simulink model "systolicArrayStreamOutput"  (R2021a)
settings: Solver=VariableStepAuto  StartTime=0.0  StopTime=13  RelTol=1e-3
libraries: hdlBasic x112, xbsIndex_r4 x1
settings Model: Creator=caval  LastModifiedBy=kv25

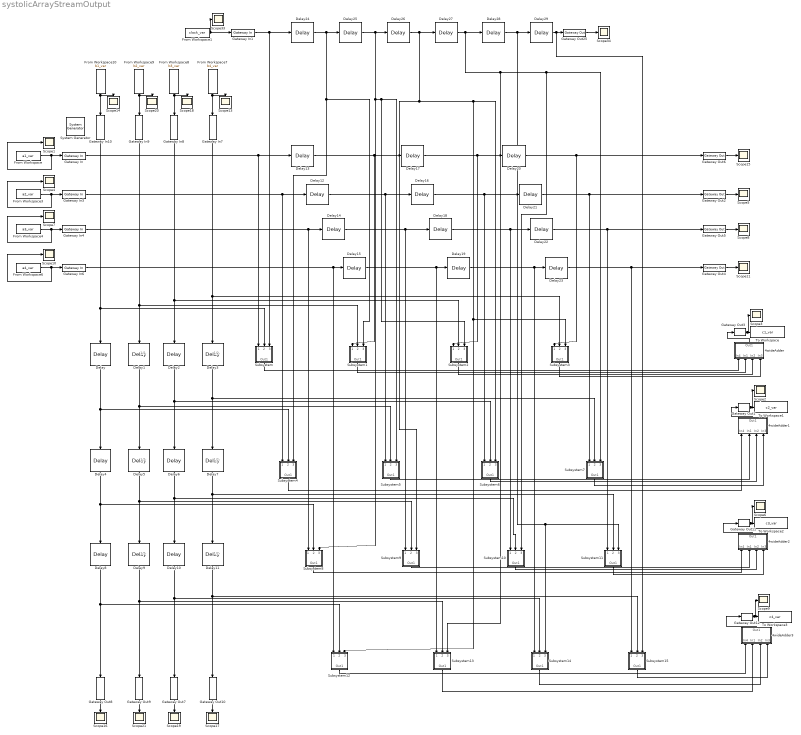
== system systolicArrayStreamOutput ==
  note: 1/2
  note: 1/2
  note: 1/2
  note: 1/2
  note: 1/2
  note: 1/2
  " System Generator" : xbsIndex_r4/ System Generator  Tag=genX  xilinxfamily=zynq  part=xc7z020  speed=-1  package=clg484  synthesis_tool=Vivado  clock_wrapper=Clock Enables  directory=./netlist2  proj_type=Vivado  Synth_file=Vivado Synthesis Defaults  Impl_file=Vivado Implementation Defaults  testbench=off  simulink_period=1  sysclk_period=10  dcm_input_clock_period=10  incr_netlist=off  trim_vbits=Everywhere in SubSystem  dbl_ovrd=According to Block Masks  core_generation=According to Block Masks  run_coregen=off  deprecated_control=off  eval_field=0  block_type=sysgen
  4wideAdder : Subsystem
  4wideAdder1 : Subsystem
  4wideAdder2 : Subsystem
  4wideAdder3 : Subsystem
  Delay{,1..29} (30 alike) : hdlBasic/Delay  rst=off  en=off  latency=1  reg_retiming=off  XmcBlockStatus=1  maskContainerNames=group1  block_type=delay  block_config=sysgen:Delay_config
  From Workspace : FromWorkspace  VariableName=a1_var
  From Workspace1 : FromWorkspace  VariableName=clock_var
  From Workspace10 : FromWorkspace  VariableName=b1_var
  From Workspace3 : FromWorkspace  VariableName=a2_var
  From Workspace4 : FromWorkspace  VariableName=a3_var
  From Workspace6 : FromWorkspace  VariableName=a4_var
  From Workspace7 : FromWorkspace  VariableName=b4_var
  From Workspace8 : FromWorkspace  VariableName=b3_var
  From Workspace9 : FromWorkspace  VariableName=b2_var
  Gateway In{,1,3..4,6..10} (9 alike) : hdlBasic/Gateway In  gui_display_data_type=Fixed-point  arith_type=Signed (2's comp)  n_bits=16  bin_pt=0  preci_type=Single  exp_width=8  frac_width=24  rows=1  columns=1  quantization="Round  (unbiased: +/- Inf)"  overflow=Saturate  period=1  UseAsADC=off  ADCChannel='1'  interface=None  automatic_assignment=on  address_offset=hex2dec('00')  intf_name=''  intf_description=''  default_value=0  timing_constraint=None  locs_specified=off  LOCs={}  io_standard={}  inherit_from_input=off  hdl_port=on  XmcBlockStatus=1  maskContainerNames=group4  block_type=gatewayin  block_config=sysgen:gateway_in_config  block_width_w=590  block_height_w=620  block_width=640  block_height=850
  Gateway Out{1..12,25} (13 alike) : hdlBasic/Gateway Out  inherit_from_input=off  hdl_port=on  rows=1  columns=1  UseAsDAC=off  DACChannel='1'  interface=None  automatic_assignment=on  address_offset=hex2dec('00')  intf_name=''  intf_description=''  timing_constraint=None  locs_specified=off  LOCs={}  io_standard={}  XmcBlockStatus=1  maskContainerNames=group4  block_type=gatewayout  block_config=sysgen:gateway_out_config  block_width_w=590  block_height_w=620  block_width=620  block_height=750
  Scope{1..11,13..21,33..34} (22 alike) : Scope
      Scope11 settings: Description=C14  AttributesFormatString=texttest
      Scope15 settings: Description=C14  AttributesFormatString=texttest
      Scope16 settings: Description=C14  AttributesFormatString=texttest
      Scope17 settings: Description=C14  AttributesFormatString=texttest
      Scope19 settings: Description=C14  AttributesFormatString=texttest
      Scope2 settings: Description=C14  AttributesFormatString=texttest
      Scope21 settings: Description=C14  AttributesFormatString=texttest
      Scope3 settings: Description=C14  AttributesFormatString=texttest
      Scope34 settings: Description=C14  AttributesFormatString=texttest
      Scope5 settings: Description=C14  AttributesFormatString=texttest
      Scope6 settings: Description=C14  AttributesFormatString=texttest
      Scope8 settings: Description=C14  AttributesFormatString=texttest
      Scope9 settings: Description=C14  AttributesFormatString=texttest
  Subsystem : Subsystem
  Subsystem1 : Subsystem
  Subsystem10 : Subsystem
  Subsystem11 : Subsystem
  Subsystem12 : Subsystem
  Subsystem13 : Subsystem
  Subsystem14 : Subsystem
  Subsystem15 : Subsystem
  Subsystem2 : Subsystem
  Subsystem3 : Subsystem
  Subsystem4 : Subsystem
  Subsystem5 : Subsystem
  Subsystem6 : Subsystem
  Subsystem7 : Subsystem
  Subsystem8 : Subsystem
  Subsystem9 : Subsystem
  To Workspace : ToWorkspace  VariableName=c1_var  SaveFormat=Timeseries  SampleTime=-1
  To Workspace1 : ToWorkspace  VariableName=c2_var  SaveFormat=Timeseries  SampleTime=-1
  To Workspace2 : ToWorkspace  VariableName=c3_var  SaveFormat=Timeseries  SampleTime=-1
  To Workspace3 : ToWorkspace  VariableName=c4_var  SaveFormat=Timeseries  SampleTime=-1
  wires:
  From Workspace/1 -> Scope1/1, Gateway In/1
  Gateway Out6/1 -> Scope15/1
  Gateway In/1 -> Delay13/1, Subsystem/1(In1)
  Gateway Out2/1 -> Scope5/1
  From Workspace3/1 -> Scope4/1, Gateway In3/1
  Gateway In3/1 -> Subsystem4/1(In1), Delay12/1
  From Workspace6/1 -> Scope10/1, Gateway In6/1
  Gateway Out5/1 -> Scope8/1
  Gateway Out4/1 -> Scope11/1
  From Workspace4/1 -> Scope7/1, Gateway In4/1
  Gateway In6/1 -> Subsystem12/1(In1), Delay15/1
  Gateway In4/1 -> Subsystem8/1(In1), Delay14/1
  From Workspace8/1 -> Scope18/1, Gateway In8/1
  Gateway Out7/1 -> Scope19/1
  Gateway In9/1 -> Subsystem1/2(In2), Delay1/1
  Gateway In10/1 -> Subsystem/2(In2), Delay/1
  Gateway Out8/1 -> Scope16/1
  From Workspace10/1 -> Scope14/1, Gateway In10/1
  Gateway Out10/1 -> Scope17/1
  From Workspace9/1 -> Scope20/1, Gateway In9/1
  Gateway Out9/1 -> Scope21/1
  From Workspace7/1 -> Scope13/1, Gateway In7/1
  Gateway In8/1 -> Subsystem2/2(In2), Delay2/1
  Gateway In7/1 -> Subsystem3/2(In2), Delay3/1
  Delay/1 -> Subsystem4/2(In2), Delay4/1
  Delay4/1 -> Subsystem8/2(In2), Delay8/1
  Delay13/1 -> Subsystem1/1(In1), Delay17/1
  Delay12/1 -> Delay16/1, Subsystem5/1(In1)
  Delay1/1 -> Subsystem5/2(In2), Delay5/1
  Delay2/1 -> Subsystem6/2(In2), Delay6/1
  Delay3/1 -> Subsystem7/2(In2), Delay7/1
  Delay5/1 -> Subsystem9/2(In2), Delay9/1
  Delay6/1 -> Subsystem10/2(In2), Delay10/1
  Delay7/1 -> Subsystem11/2(In2), Delay11/1
  Delay20/1 -> Subsystem3/1(In1), Gateway Out6/1
  Delay16/1 -> Subsystem6/1(In1), Delay21/1
  Delay21/1 -> Subsystem7/1(In1), Gateway Out2/1
  Delay8/1 -> Subsystem12/2(In2), Gateway Out8/1
  Delay11/1 -> Subsystem15/2(In2), Gateway Out10/1
  Delay9/1 -> Subsystem13/2(In2), Gateway Out9/1
  Delay10/1 -> Subsystem14/2(In2), Gateway Out7/1
  Delay18/1 -> Subsystem10/1(In1), Delay22/1
  Delay22/1 -> Subsystem11/1(In1), Gateway Out5/1
  Delay19/1 -> Subsystem14/1(In1), Delay23/1
  Delay23/1 -> Subsystem15/1(In1), Gateway Out4/1
  Delay14/1 -> Subsystem9/1(In1), Delay18/1
  Delay15/1 -> Subsystem13/1(In1), Delay19/1
  Delay17/1 -> Subsystem2/1(In1), Delay20/1
  From Workspace1/1 -> Scope33/1, Gateway In1/1
  Gateway In1/1 -> Subsystem/3(In3), Delay24/1
  Delay24/1 -> Subsystem4/3(In3), Subsystem1/3(In3), Delay25/1
  Delay25/1 -> Subsystem8/3(In3), Subsystem5/3(In3), Subsystem2/3(In3), Delay26/1
  Delay28/1 -> Delay29/1, Subsystem14/3(In3), Subsystem11/3(In3)
  Delay27/1 -> Subsystem13/3(In3), Subsystem10/3(In3), Subsystem7/3(In3), Delay28/1
  Gateway Out25/1 -> Scope34/1
  Delay29/1 -> Subsystem15/3(In3), Gateway Out25/1
  Delay26/1 -> Subsystem9/3(In3), Subsystem6/3(In3), Subsystem12/3(In3), Subsystem3/3(In3), Delay27/1
  4wideAdder/1(Out1) -> Gateway Out3/1
  Gateway Out3/1 -> Scope3/1, To Workspace/1
  Subsystem1/1(Out1) -> 4wideAdder/2(In1)
  Subsystem2/1(Out1) -> 4wideAdder/3(In2)
  Subsystem3/1(Out1) -> 4wideAdder/4(In3)
  Subsystem4/1(Out1) -> 4wideAdder1/1(In4)
  Subsystem5/1(Out1) -> 4wideAdder1/2(In1)
  Subsystem6/1(Out1) -> 4wideAdder1/3(In2)
  Subsystem7/1(Out1) -> 4wideAdder1/4(In3)
  Subsystem8/1(Out1) -> 4wideAdder2/1(In4)
  Subsystem9/1(Out1) -> 4wideAdder2/2(In1)
  Subsystem10/1(Out1) -> 4wideAdder2/3(In2)
  Subsystem11/1(Out1) -> 4wideAdder2/4(In3)
  Subsystem12/1(Out1) -> 4wideAdder3/1(In4)
  Subsystem13/1(Out1) -> 4wideAdder3/2(In1)
  Subsystem14/1(Out1) -> 4wideAdder3/3(In2)
  Subsystem15/1(Out1) -> 4wideAdder3/4(In3)
  Subsystem/1(Out1) -> 4wideAdder/1(In4)
  4wideAdder1/1(Out1) -> Gateway Out1/1
  Gateway Out1/1 -> Scope2/1, To Workspace1/1
  4wideAdder2/1(Out1) -> Gateway Out11/1
  Gateway Out11/1 -> Scope6/1, To Workspace2/1
  4wideAdder3/1(Out1) -> Gateway Out12/1
  Gateway Out12/1 -> Scope9/1, To Workspace3/1

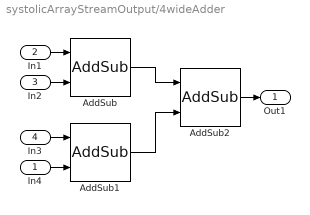
== system systolicArrayStreamOutput/4wideAdder ==
  In4 : Inport
  In1 : Inport  Port=2
  In2 : Inport  Port=3
  In3 : Inport  Port=4
  AddSub : hdlBasic/AddSub  mode=Addition  use_carryin=off  use_carryout=off  en=off  latency=0  precision=Full  arith_type=Unsigned  n_bits=16  bin_pt=14  quantization=Truncate  overflow=Wrap  use_behavioral_HDL=off  hw_selection=Fabric  pipelined=off  XmcBlockStatus=1  maskContainerNames=tabcontainer1  block_type=addsub  block_config=sysgen:Addsub_config
  AddSub1 : hdlBasic/AddSub  mode=Addition  use_carryin=off  use_carryout=off  en=off  latency=0  precision=Full  arith_type=Unsigned  n_bits=16  bin_pt=14  quantization=Truncate  overflow=Wrap  use_behavioral_HDL=off  hw_selection=Fabric  pipelined=off  XmcBlockStatus=1  maskContainerNames=tabcontainer1  block_type=addsub  block_config=sysgen:Addsub_config
  AddSub2 : hdlBasic/AddSub  mode=Addition  use_carryin=off  use_carryout=off  en=off  latency=0  precision=Full  arith_type=Unsigned  n_bits=16  bin_pt=14  quantization=Truncate  overflow=Wrap  use_behavioral_HDL=off  hw_selection=Fabric  pipelined=off  XmcBlockStatus=1  maskContainerNames=tabcontainer1  block_type=addsub  block_config=sysgen:Addsub_config
  Out1 : Outport
  wires:
  In1/1 -> AddSub/1
  AddSub1/1 -> AddSub2/2
  AddSub/1 -> AddSub2/1
  In4/1 -> AddSub1/2
  In3/1 -> AddSub1/1
  AddSub2/1 -> Out1/1
  In2/1 -> AddSub/2

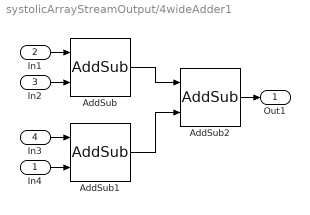
== system systolicArrayStreamOutput/4wideAdder1 ==
  In4 : Inport
  In1 : Inport  Port=2
  In2 : Inport  Port=3
  In3 : Inport  Port=4
  AddSub : hdlBasic/AddSub  mode=Addition  use_carryin=off  use_carryout=off  en=off  latency=0  precision=Full  arith_type=Unsigned  n_bits=16  bin_pt=14  quantization=Truncate  overflow=Wrap  use_behavioral_HDL=off  hw_selection=Fabric  pipelined=off  XmcBlockStatus=1  maskContainerNames=tabcontainer1  block_type=addsub  block_config=sysgen:Addsub_config
  AddSub1 : hdlBasic/AddSub  mode=Addition  use_carryin=off  use_carryout=off  en=off  latency=0  precision=Full  arith_type=Unsigned  n_bits=16  bin_pt=14  quantization=Truncate  overflow=Wrap  use_behavioral_HDL=off  hw_selection=Fabric  pipelined=off  XmcBlockStatus=1  maskContainerNames=tabcontainer1  block_type=addsub  block_config=sysgen:Addsub_config
  AddSub2 : hdlBasic/AddSub  mode=Addition  use_carryin=off  use_carryout=off  en=off  latency=0  precision=Full  arith_type=Unsigned  n_bits=16  bin_pt=14  quantization=Truncate  overflow=Wrap  use_behavioral_HDL=off  hw_selection=Fabric  pipelined=off  XmcBlockStatus=1  maskContainerNames=tabcontainer1  block_type=addsub  block_config=sysgen:Addsub_config
  Out1 : Outport
  wires:
  In1/1 -> AddSub/1
  AddSub1/1 -> AddSub2/2
  AddSub/1 -> AddSub2/1
  In4/1 -> AddSub1/2
  In3/1 -> AddSub1/1
  AddSub2/1 -> Out1/1
  In2/1 -> AddSub/2

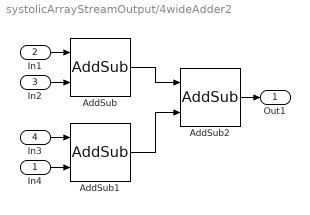
== system systolicArrayStreamOutput/4wideAdder2 ==
  In4 : Inport
  In1 : Inport  Port=2
  In2 : Inport  Port=3
  In3 : Inport  Port=4
  AddSub : hdlBasic/AddSub  mode=Addition  use_carryin=off  use_carryout=off  en=off  latency=0  precision=Full  arith_type=Unsigned  n_bits=16  bin_pt=14  quantization=Truncate  overflow=Wrap  use_behavioral_HDL=off  hw_selection=Fabric  pipelined=off  XmcBlockStatus=1  maskContainerNames=tabcontainer1  block_type=addsub  block_config=sysgen:Addsub_config
  AddSub1 : hdlBasic/AddSub  mode=Addition  use_carryin=off  use_carryout=off  en=off  latency=0  precision=Full  arith_type=Unsigned  n_bits=16  bin_pt=14  quantization=Truncate  overflow=Wrap  use_behavioral_HDL=off  hw_selection=Fabric  pipelined=off  XmcBlockStatus=1  maskContainerNames=tabcontainer1  block_type=addsub  block_config=sysgen:Addsub_config
  AddSub2 : hdlBasic/AddSub  mode=Addition  use_carryin=off  use_carryout=off  en=off  latency=0  precision=Full  arith_type=Unsigned  n_bits=16  bin_pt=14  quantization=Truncate  overflow=Wrap  use_behavioral_HDL=off  hw_selection=Fabric  pipelined=off  XmcBlockStatus=1  maskContainerNames=tabcontainer1  block_type=addsub  block_config=sysgen:Addsub_config
  Out1 : Outport
  wires:
  In1/1 -> AddSub/1
  AddSub1/1 -> AddSub2/2
  AddSub/1 -> AddSub2/1
  In4/1 -> AddSub1/2
  In3/1 -> AddSub1/1
  AddSub2/1 -> Out1/1
  In2/1 -> AddSub/2

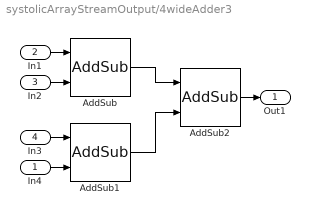
== system systolicArrayStreamOutput/4wideAdder3 ==
  In4 : Inport
  In1 : Inport  Port=2
  In2 : Inport  Port=3
  In3 : Inport  Port=4
  AddSub : hdlBasic/AddSub  mode=Addition  use_carryin=off  use_carryout=off  en=off  latency=0  precision=Full  arith_type=Unsigned  n_bits=16  bin_pt=14  quantization=Truncate  overflow=Wrap  use_behavioral_HDL=off  hw_selection=Fabric  pipelined=off  XmcBlockStatus=1  maskContainerNames=tabcontainer1  block_type=addsub  block_config=sysgen:Addsub_config
  AddSub1 : hdlBasic/AddSub  mode=Addition  use_carryin=off  use_carryout=off  en=off  latency=0  precision=Full  arith_type=Unsigned  n_bits=16  bin_pt=14  quantization=Truncate  overflow=Wrap  use_behavioral_HDL=off  hw_selection=Fabric  pipelined=off  XmcBlockStatus=1  maskContainerNames=tabcontainer1  block_type=addsub  block_config=sysgen:Addsub_config
  AddSub2 : hdlBasic/AddSub  mode=Addition  use_carryin=off  use_carryout=off  en=off  latency=0  precision=Full  arith_type=Unsigned  n_bits=16  bin_pt=14  quantization=Truncate  overflow=Wrap  use_behavioral_HDL=off  hw_selection=Fabric  pipelined=off  XmcBlockStatus=1  maskContainerNames=tabcontainer1  block_type=addsub  block_config=sysgen:Addsub_config
  Out1 : Outport
  wires:
  In1/1 -> AddSub/1
  AddSub1/1 -> AddSub2/2
  AddSub/1 -> AddSub2/1
  In4/1 -> AddSub1/2
  In3/1 -> AddSub1/1
  AddSub2/1 -> Out1/1
  In2/1 -> AddSub/2

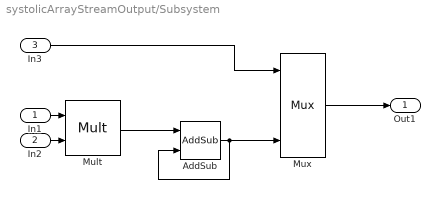
== system systolicArrayStreamOutput/Subsystem ==
  In1 : Inport
  In2 : Inport  Port=2
  In3 : Inport  Port=3
  AddSub : hdlBasic/AddSub  mode=Addition  use_carryin=off  use_carryout=off  en=off  latency=1  precision=User Defined  arith_type=Unsigned  n_bits=16  bin_pt=0  quantization=Truncate  overflow=Wrap  use_behavioral_HDL=off  hw_selection=Fabric  pipelined=off  XmcBlockStatus=1  maskContainerNames=tabcontainer1  block_type=addsub  block_config=sysgen:Addsub_config
  Mult : hdlBasic/Mult  precision=Full  arith_type="Signed  (2's comp)"  n_bits=16  bin_pt=14  quantization=Truncate  overflow=Wrap  en=off  latency=0  use_behavioral_HDL=off  opt=Speed  use_embedded=on  optimum_pipeline=off  pipeline=on  use_rpm=on  placement_style=Triangular  XmcBlockStatus=1  maskContainerNames=group1  block_type=mult  block_config=sysgen:Mult_config
  Mux : hdlBasic/Mux  inputs=2  en=off  latency=1  precision=Full  arith_type=Unsigned  n_bits=16  bin_pt=14  quantization=Truncate  overflow=Wrap  XmcBlockStatus=1  maskContainerNames=tabcontainer1  block_type=mux  block_config=sysgen:Mux_config
  Out1 : Outport
  wires:
  In1/1 -> Mult/1
  AddSub/1 -> Mux/3, AddSub/2
  In2/1 -> Mult/2
  Mult/1 -> AddSub/1
  In3/1 -> Mux/1
  Mux/1 -> Out1/1

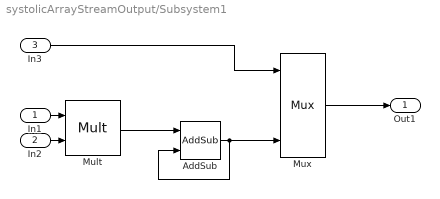
== system systolicArrayStreamOutput/Subsystem1 ==
  In1 : Inport
  In2 : Inport  Port=2
  In3 : Inport  Port=3
  AddSub : hdlBasic/AddSub  mode=Addition  use_carryin=off  use_carryout=off  en=off  latency=1  precision=User Defined  arith_type=Unsigned  n_bits=16  bin_pt=0  quantization=Truncate  overflow=Wrap  use_behavioral_HDL=off  hw_selection=Fabric  pipelined=off  XmcBlockStatus=1  maskContainerNames=tabcontainer1  block_type=addsub  block_config=sysgen:Addsub_config
  Mult : hdlBasic/Mult  precision=Full  arith_type="Signed  (2's comp)"  n_bits=16  bin_pt=14  quantization=Truncate  overflow=Wrap  en=off  latency=0  use_behavioral_HDL=off  opt=Speed  use_embedded=on  optimum_pipeline=off  pipeline=on  use_rpm=on  placement_style=Triangular  XmcBlockStatus=1  maskContainerNames=group1  block_type=mult  block_config=sysgen:Mult_config
  Mux : hdlBasic/Mux  inputs=2  en=off  latency=1  precision=Full  arith_type=Unsigned  n_bits=16  bin_pt=14  quantization=Truncate  overflow=Wrap  XmcBlockStatus=1  maskContainerNames=tabcontainer1  block_type=mux  block_config=sysgen:Mux_config
  Out1 : Outport
  wires:
  In1/1 -> Mult/1
  AddSub/1 -> Mux/3, AddSub/2
  In2/1 -> Mult/2
  Mult/1 -> AddSub/1
  In3/1 -> Mux/1
  Mux/1 -> Out1/1

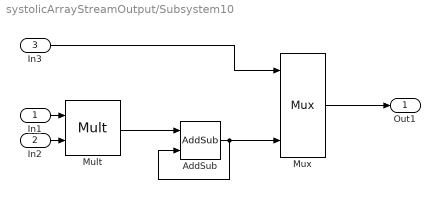
== system systolicArrayStreamOutput/Subsystem10 ==
  In1 : Inport
  In2 : Inport  Port=2
  In3 : Inport  Port=3
  AddSub : hdlBasic/AddSub  mode=Addition  use_carryin=off  use_carryout=off  en=off  latency=1  precision=User Defined  arith_type=Unsigned  n_bits=16  bin_pt=0  quantization=Truncate  overflow=Wrap  use_behavioral_HDL=off  hw_selection=Fabric  pipelined=off  XmcBlockStatus=1  maskContainerNames=tabcontainer1  block_type=addsub  block_config=sysgen:Addsub_config
  Mult : hdlBasic/Mult  precision=Full  arith_type="Signed  (2's comp)"  n_bits=16  bin_pt=14  quantization=Truncate  overflow=Wrap  en=off  latency=0  use_behavioral_HDL=off  opt=Speed  use_embedded=on  optimum_pipeline=off  pipeline=on  use_rpm=on  placement_style=Triangular  XmcBlockStatus=1  maskContainerNames=group1  block_type=mult  block_config=sysgen:Mult_config
  Mux : hdlBasic/Mux  inputs=2  en=off  latency=1  precision=Full  arith_type=Unsigned  n_bits=16  bin_pt=14  quantization=Truncate  overflow=Wrap  XmcBlockStatus=1  maskContainerNames=tabcontainer1  block_type=mux  block_config=sysgen:Mux_config
  Out1 : Outport
  wires:
  In1/1 -> Mult/1
  AddSub/1 -> Mux/3, AddSub/2
  In2/1 -> Mult/2
  Mult/1 -> AddSub/1
  In3/1 -> Mux/1
  Mux/1 -> Out1/1

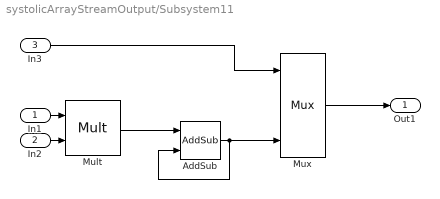
== system systolicArrayStreamOutput/Subsystem11 ==
  In1 : Inport
  In2 : Inport  Port=2
  In3 : Inport  Port=3
  AddSub : hdlBasic/AddSub  mode=Addition  use_carryin=off  use_carryout=off  en=off  latency=1  precision=User Defined  arith_type=Unsigned  n_bits=16  bin_pt=0  quantization=Truncate  overflow=Wrap  use_behavioral_HDL=off  hw_selection=Fabric  pipelined=off  XmcBlockStatus=1  maskContainerNames=tabcontainer1  block_type=addsub  block_config=sysgen:Addsub_config
  Mult : hdlBasic/Mult  precision=Full  arith_type="Signed  (2's comp)"  n_bits=16  bin_pt=14  quantization=Truncate  overflow=Wrap  en=off  latency=0  use_behavioral_HDL=off  opt=Speed  use_embedded=on  optimum_pipeline=off  pipeline=on  use_rpm=on  placement_style=Triangular  XmcBlockStatus=1  maskContainerNames=group1  block_type=mult  block_config=sysgen:Mult_config
  Mux : hdlBasic/Mux  inputs=2  en=off  latency=1  precision=Full  arith_type=Unsigned  n_bits=16  bin_pt=14  quantization=Truncate  overflow=Wrap  XmcBlockStatus=1  maskContainerNames=tabcontainer1  block_type=mux  block_config=sysgen:Mux_config
  Out1 : Outport
  wires:
  In1/1 -> Mult/1
  AddSub/1 -> Mux/3, AddSub/2
  In2/1 -> Mult/2
  Mult/1 -> AddSub/1
  In3/1 -> Mux/1
  Mux/1 -> Out1/1

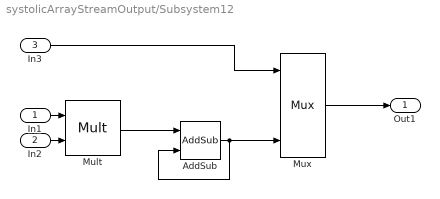
== system systolicArrayStreamOutput/Subsystem12 ==
  In1 : Inport
  In2 : Inport  Port=2
  In3 : Inport  Port=3
  AddSub : hdlBasic/AddSub  mode=Addition  use_carryin=off  use_carryout=off  en=off  latency=1  precision=User Defined  arith_type=Unsigned  n_bits=16  bin_pt=0  quantization=Truncate  overflow=Wrap  use_behavioral_HDL=off  hw_selection=Fabric  pipelined=off  XmcBlockStatus=1  maskContainerNames=tabcontainer1  block_type=addsub  block_config=sysgen:Addsub_config
  Mult : hdlBasic/Mult  precision=Full  arith_type="Signed  (2's comp)"  n_bits=16  bin_pt=14  quantization=Truncate  overflow=Wrap  en=off  latency=0  use_behavioral_HDL=off  opt=Speed  use_embedded=on  optimum_pipeline=off  pipeline=on  use_rpm=on  placement_style=Triangular  XmcBlockStatus=1  maskContainerNames=group1  block_type=mult  block_config=sysgen:Mult_config
  Mux : hdlBasic/Mux  inputs=2  en=off  latency=1  precision=Full  arith_type=Unsigned  n_bits=16  bin_pt=14  quantization=Truncate  overflow=Wrap  XmcBlockStatus=1  maskContainerNames=tabcontainer1  block_type=mux  block_config=sysgen:Mux_config
  Out1 : Outport
  wires:
  In1/1 -> Mult/1
  AddSub/1 -> Mux/3, AddSub/2
  In2/1 -> Mult/2
  Mult/1 -> AddSub/1
  In3/1 -> Mux/1
  Mux/1 -> Out1/1

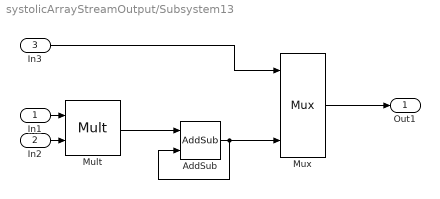
== system systolicArrayStreamOutput/Subsystem13 ==
  In1 : Inport
  In2 : Inport  Port=2
  In3 : Inport  Port=3
  AddSub : hdlBasic/AddSub  mode=Addition  use_carryin=off  use_carryout=off  en=off  latency=1  precision=User Defined  arith_type=Unsigned  n_bits=16  bin_pt=0  quantization=Truncate  overflow=Wrap  use_behavioral_HDL=off  hw_selection=Fabric  pipelined=off  XmcBlockStatus=1  maskContainerNames=tabcontainer1  block_type=addsub  block_config=sysgen:Addsub_config
  Mult : hdlBasic/Mult  precision=Full  arith_type="Signed  (2's comp)"  n_bits=16  bin_pt=14  quantization=Truncate  overflow=Wrap  en=off  latency=0  use_behavioral_HDL=off  opt=Speed  use_embedded=on  optimum_pipeline=off  pipeline=on  use_rpm=on  placement_style=Triangular  XmcBlockStatus=1  maskContainerNames=group1  block_type=mult  block_config=sysgen:Mult_config
  Mux : hdlBasic/Mux  inputs=2  en=off  latency=1  precision=Full  arith_type=Unsigned  n_bits=16  bin_pt=14  quantization=Truncate  overflow=Wrap  XmcBlockStatus=1  maskContainerNames=tabcontainer1  block_type=mux  block_config=sysgen:Mux_config
  Out1 : Outport
  wires:
  In1/1 -> Mult/1
  AddSub/1 -> Mux/3, AddSub/2
  In2/1 -> Mult/2
  Mult/1 -> AddSub/1
  In3/1 -> Mux/1
  Mux/1 -> Out1/1

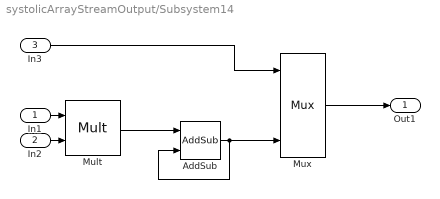
== system systolicArrayStreamOutput/Subsystem14 ==
  In1 : Inport
  In2 : Inport  Port=2
  In3 : Inport  Port=3
  AddSub : hdlBasic/AddSub  mode=Addition  use_carryin=off  use_carryout=off  en=off  latency=1  precision=User Defined  arith_type=Unsigned  n_bits=16  bin_pt=0  quantization=Truncate  overflow=Wrap  use_behavioral_HDL=off  hw_selection=Fabric  pipelined=off  XmcBlockStatus=1  maskContainerNames=tabcontainer1  block_type=addsub  block_config=sysgen:Addsub_config
  Mult : hdlBasic/Mult  precision=Full  arith_type="Signed  (2's comp)"  n_bits=16  bin_pt=14  quantization=Truncate  overflow=Wrap  en=off  latency=0  use_behavioral_HDL=off  opt=Speed  use_embedded=on  optimum_pipeline=off  pipeline=on  use_rpm=on  placement_style=Triangular  XmcBlockStatus=1  maskContainerNames=group1  block_type=mult  block_config=sysgen:Mult_config
  Mux : hdlBasic/Mux  inputs=2  en=off  latency=1  precision=Full  arith_type=Unsigned  n_bits=16  bin_pt=14  quantization=Truncate  overflow=Wrap  XmcBlockStatus=1  maskContainerNames=tabcontainer1  block_type=mux  block_config=sysgen:Mux_config
  Out1 : Outport
  wires:
  In1/1 -> Mult/1
  AddSub/1 -> Mux/3, AddSub/2
  In2/1 -> Mult/2
  Mult/1 -> AddSub/1
  In3/1 -> Mux/1
  Mux/1 -> Out1/1

== system systolicArrayStreamOutput/Subsystem15 ==
  In1 : Inport
  In2 : Inport  Port=2
  In3 : Inport  Port=3
  AddSub : hdlBasic/AddSub  mode=Addition  use_carryin=off  use_carryout=off  en=off  latency=1  precision=User Defined  arith_type=Unsigned  n_bits=16  bin_pt=0  quantization=Truncate  overflow=Wrap  use_behavioral_HDL=off  hw_selection=Fabric  pipelined=off  XmcBlockStatus=1  maskContainerNames=tabcontainer1  block_type=addsub  block_config=sysgen:Addsub_config
  Mult : hdlBasic/Mult  precision=Full  arith_type="Signed  (2's comp)"  n_bits=16  bin_pt=14  quantization=Truncate  overflow=Wrap  en=off  latency=0  use_behavioral_HDL=off  opt=Speed  use_embedded=on  optimum_pipeline=off  pipeline=on  use_rpm=on  placement_style=Triangular  XmcBlockStatus=1  maskContainerNames=group1  block_type=mult  block_config=sysgen:Mult_config
  Mux : hdlBasic/Mux  inputs=2  en=off  latency=1  precision=Full  arith_type=Unsigned  n_bits=16  bin_pt=14  quantization=Truncate  overflow=Wrap  XmcBlockStatus=1  maskContainerNames=tabcontainer1  block_type=mux  block_config=sysgen:Mux_config
  Out1 : Outport
  wires:
  In1/1 -> Mult/1
  AddSub/1 -> Mux/3, AddSub/2
  In2/1 -> Mult/2
  Mult/1 -> AddSub/1
  In3/1 -> Mux/1
  Mux/1 -> Out1/1

== system systolicArrayStreamOutput/Subsystem2 ==
  In1 : Inport
  In2 : Inport  Port=2
  In3 : Inport  Port=3
  AddSub : hdlBasic/AddSub  mode=Addition  use_carryin=off  use_carryout=off  en=off  latency=1  precision=User Defined  arith_type=Unsigned  n_bits=16  bin_pt=0  quantization=Truncate  overflow=Wrap  use_behavioral_HDL=off  hw_selection=Fabric  pipelined=off  XmcBlockStatus=1  maskContainerNames=tabcontainer1  block_type=addsub  block_config=sysgen:Addsub_config
  Mult : hdlBasic/Mult  precision=Full  arith_type="Signed  (2's comp)"  n_bits=16  bin_pt=14  quantization=Truncate  overflow=Wrap  en=off  latency=0  use_behavioral_HDL=off  opt=Speed  use_embedded=on  optimum_pipeline=off  pipeline=on  use_rpm=on  placement_style=Triangular  XmcBlockStatus=1  maskContainerNames=group1  block_type=mult  block_config=sysgen:Mult_config
  Mux : hdlBasic/Mux  inputs=2  en=off  latency=1  precision=Full  arith_type=Unsigned  n_bits=16  bin_pt=14  quantization=Truncate  overflow=Wrap  XmcBlockStatus=1  maskContainerNames=tabcontainer1  block_type=mux  block_config=sysgen:Mux_config
  Out1 : Outport
  wires:
  In1/1 -> Mult/1
  AddSub/1 -> Mux/3, AddSub/2
  In2/1 -> Mult/2
  Mult/1 -> AddSub/1
  In3/1 -> Mux/1
  Mux/1 -> Out1/1

== system systolicArrayStreamOutput/Subsystem3 ==
  In1 : Inport
  In2 : Inport  Port=2
  In3 : Inport  Port=3
  AddSub : hdlBasic/AddSub  mode=Addition  use_carryin=off  use_carryout=off  en=off  latency=1  precision=User Defined  arith_type=Unsigned  n_bits=16  bin_pt=0  quantization=Truncate  overflow=Wrap  use_behavioral_HDL=off  hw_selection=Fabric  pipelined=off  XmcBlockStatus=1  maskContainerNames=tabcontainer1  block_type=addsub  block_config=sysgen:Addsub_config
  Mult : hdlBasic/Mult  precision=Full  arith_type="Signed  (2's comp)"  n_bits=16  bin_pt=14  quantization=Truncate  overflow=Wrap  en=off  latency=0  use_behavioral_HDL=off  opt=Speed  use_embedded=on  optimum_pipeline=off  pipeline=on  use_rpm=on  placement_style=Triangular  XmcBlockStatus=1  maskContainerNames=group1  block_type=mult  block_config=sysgen:Mult_config
  Mux : hdlBasic/Mux  inputs=2  en=off  latency=1  precision=Full  arith_type=Unsigned  n_bits=16  bin_pt=14  quantization=Truncate  overflow=Wrap  XmcBlockStatus=1  maskContainerNames=tabcontainer1  block_type=mux  block_config=sysgen:Mux_config
  Out1 : Outport
  wires:
  In1/1 -> Mult/1
  AddSub/1 -> Mux/3, AddSub/2
  In2/1 -> Mult/2
  Mult/1 -> AddSub/1
  In3/1 -> Mux/1
  Mux/1 -> Out1/1

== system systolicArrayStreamOutput/Subsystem4 ==
  In1 : Inport
  In2 : Inport  Port=2
  In3 : Inport  Port=3
  AddSub : hdlBasic/AddSub  mode=Addition  use_carryin=off  use_carryout=off  en=off  latency=1  precision=User Defined  arith_type=Unsigned  n_bits=16  bin_pt=0  quantization=Truncate  overflow=Wrap  use_behavioral_HDL=off  hw_selection=Fabric  pipelined=off  XmcBlockStatus=1  maskContainerNames=tabcontainer1  block_type=addsub  block_config=sysgen:Addsub_config
  Mult : hdlBasic/Mult  precision=Full  arith_type="Signed  (2's comp)"  n_bits=16  bin_pt=14  quantization=Truncate  overflow=Wrap  en=off  latency=0  use_behavioral_HDL=off  opt=Speed  use_embedded=on  optimum_pipeline=off  pipeline=on  use_rpm=on  placement_style=Triangular  XmcBlockStatus=1  maskContainerNames=group1  block_type=mult  block_config=sysgen:Mult_config
  Mux : hdlBasic/Mux  inputs=2  en=off  latency=1  precision=Full  arith_type=Unsigned  n_bits=16  bin_pt=14  quantization=Truncate  overflow=Wrap  XmcBlockStatus=1  maskContainerNames=tabcontainer1  block_type=mux  block_config=sysgen:Mux_config
  Out1 : Outport
  wires:
  In1/1 -> Mult/1
  AddSub/1 -> Mux/3, AddSub/2
  In2/1 -> Mult/2
  Mult/1 -> AddSub/1
  In3/1 -> Mux/1
  Mux/1 -> Out1/1

== system systolicArrayStreamOutput/Subsystem5 ==
  In1 : Inport
  In2 : Inport  Port=2
  In3 : Inport  Port=3
  AddSub : hdlBasic/AddSub  mode=Addition  use_carryin=off  use_carryout=off  en=off  latency=1  precision=User Defined  arith_type=Unsigned  n_bits=16  bin_pt=0  quantization=Truncate  overflow=Wrap  use_behavioral_HDL=off  hw_selection=Fabric  pipelined=off  XmcBlockStatus=1  maskContainerNames=tabcontainer1  block_type=addsub  block_config=sysgen:Addsub_config
  Mult : hdlBasic/Mult  precision=Full  arith_type="Signed  (2's comp)"  n_bits=16  bin_pt=14  quantization=Truncate  overflow=Wrap  en=off  latency=0  use_behavioral_HDL=off  opt=Speed  use_embedded=on  optimum_pipeline=off  pipeline=on  use_rpm=on  placement_style=Triangular  XmcBlockStatus=1  maskContainerNames=group1  block_type=mult  block_config=sysgen:Mult_config
  Mux : hdlBasic/Mux  inputs=2  en=off  latency=1  precision=Full  arith_type=Unsigned  n_bits=16  bin_pt=14  quantization=Truncate  overflow=Wrap  XmcBlockStatus=1  maskContainerNames=tabcontainer1  block_type=mux  block_config=sysgen:Mux_config
  Out1 : Outport
  wires:
  In1/1 -> Mult/1
  AddSub/1 -> Mux/3, AddSub/2
  In2/1 -> Mult/2
  Mult/1 -> AddSub/1
  In3/1 -> Mux/1
  Mux/1 -> Out1/1

== system systolicArrayStreamOutput/Subsystem6 ==
  In1 : Inport
  In2 : Inport  Port=2
  In3 : Inport  Port=3
  AddSub : hdlBasic/AddSub  mode=Addition  use_carryin=off  use_carryout=off  en=off  latency=1  precision=User Defined  arith_type=Unsigned  n_bits=16  bin_pt=0  quantization=Truncate  overflow=Wrap  use_behavioral_HDL=off  hw_selection=Fabric  pipelined=off  XmcBlockStatus=1  maskContainerNames=tabcontainer1  block_type=addsub  block_config=sysgen:Addsub_config
  Mult : hdlBasic/Mult  precision=Full  arith_type="Signed  (2's comp)"  n_bits=16  bin_pt=14  quantization=Truncate  overflow=Wrap  en=off  latency=0  use_behavioral_HDL=off  opt=Speed  use_embedded=on  optimum_pipeline=off  pipeline=on  use_rpm=on  placement_style=Triangular  XmcBlockStatus=1  maskContainerNames=group1  block_type=mult  block_config=sysgen:Mult_config
  Mux : hdlBasic/Mux  inputs=2  en=off  latency=1  precision=Full  arith_type=Unsigned  n_bits=16  bin_pt=14  quantization=Truncate  overflow=Wrap  XmcBlockStatus=1  maskContainerNames=tabcontainer1  block_type=mux  block_config=sysgen:Mux_config
  Out1 : Outport
  wires:
  In1/1 -> Mult/1
  AddSub/1 -> Mux/3, AddSub/2
  In2/1 -> Mult/2
  Mult/1 -> AddSub/1
  In3/1 -> Mux/1
  Mux/1 -> Out1/1

== system systolicArrayStreamOutput/Subsystem7 ==
  In1 : Inport
  In2 : Inport  Port=2
  In3 : Inport  Port=3
  AddSub : hdlBasic/AddSub  mode=Addition  use_carryin=off  use_carryout=off  en=off  latency=1  precision=User Defined  arith_type=Unsigned  n_bits=16  bin_pt=0  quantization=Truncate  overflow=Wrap  use_behavioral_HDL=off  hw_selection=Fabric  pipelined=off  XmcBlockStatus=1  maskContainerNames=tabcontainer1  block_type=addsub  block_config=sysgen:Addsub_config
  Mult : hdlBasic/Mult  precision=Full  arith_type="Signed  (2's comp)"  n_bits=16  bin_pt=14  quantization=Truncate  overflow=Wrap  en=off  latency=0  use_behavioral_HDL=off  opt=Speed  use_embedded=on  optimum_pipeline=off  pipeline=on  use_rpm=on  placement_style=Triangular  XmcBlockStatus=1  maskContainerNames=group1  block_type=mult  block_config=sysgen:Mult_config
  Mux : hdlBasic/Mux  inputs=2  en=off  latency=1  precision=Full  arith_type=Unsigned  n_bits=16  bin_pt=14  quantization=Truncate  overflow=Wrap  XmcBlockStatus=1  maskContainerNames=tabcontainer1  block_type=mux  block_config=sysgen:Mux_config
  Out1 : Outport
  wires:
  In1/1 -> Mult/1
  AddSub/1 -> Mux/3, AddSub/2
  In2/1 -> Mult/2
  Mult/1 -> AddSub/1
  In3/1 -> Mux/1
  Mux/1 -> Out1/1

== system systolicArrayStreamOutput/Subsystem8 ==
  In1 : Inport
  In2 : Inport  Port=2
  In3 : Inport  Port=3
  AddSub : hdlBasic/AddSub  mode=Addition  use_carryin=off  use_carryout=off  en=off  latency=1  precision=User Defined  arith_type=Unsigned  n_bits=16  bin_pt=0  quantization=Truncate  overflow=Wrap  use_behavioral_HDL=off  hw_selection=Fabric  pipelined=off  XmcBlockStatus=1  maskContainerNames=tabcontainer1  block_type=addsub  block_config=sysgen:Addsub_config
  Mult : hdlBasic/Mult  precision=Full  arith_type="Signed  (2's comp)"  n_bits=16  bin_pt=14  quantization=Truncate  overflow=Wrap  en=off  latency=0  use_behavioral_HDL=off  opt=Speed  use_embedded=on  optimum_pipeline=off  pipeline=on  use_rpm=on  placement_style=Triangular  XmcBlockStatus=1  maskContainerNames=group1  block_type=mult  block_config=sysgen:Mult_config
  Mux : hdlBasic/Mux  inputs=2  en=off  latency=1  precision=Full  arith_type=Unsigned  n_bits=16  bin_pt=14  quantization=Truncate  overflow=Wrap  XmcBlockStatus=1  maskContainerNames=tabcontainer1  block_type=mux  block_config=sysgen:Mux_config
  Out1 : Outport
  wires:
  In1/1 -> Mult/1
  AddSub/1 -> Mux/3, AddSub/2
  In2/1 -> Mult/2
  Mult/1 -> AddSub/1
  In3/1 -> Mux/1
  Mux/1 -> Out1/1

== system systolicArrayStreamOutput/Subsystem9 ==
  In1 : Inport
  In2 : Inport  Port=2
  In3 : Inport  Port=3
  AddSub : hdlBasic/AddSub  mode=Addition  use_carryin=off  use_carryout=off  en=off  latency=1  precision=User Defined  arith_type=Unsigned  n_bits=16  bin_pt=0  quantization=Truncate  overflow=Wrap  use_behavioral_HDL=off  hw_selection=Fabric  pipelined=off  XmcBlockStatus=1  maskContainerNames=tabcontainer1  block_type=addsub  block_config=sysgen:Addsub_config
  Mult : hdlBasic/Mult  precision=Full  arith_type="Signed  (2's comp)"  n_bits=16  bin_pt=14  quantization=Truncate  overflow=Wrap  en=off  latency=0  use_behavioral_HDL=off  opt=Speed  use_embedded=on  optimum_pipeline=off  pipeline=on  use_rpm=on  placement_style=Triangular  XmcBlockStatus=1  maskContainerNames=group1  block_type=mult  block_config=sysgen:Mult_config
  Mux : hdlBasic/Mux  inputs=2  en=off  latency=1  precision=Full  arith_type=Unsigned  n_bits=16  bin_pt=14  quantization=Truncate  overflow=Wrap  XmcBlockStatus=1  maskContainerNames=tabcontainer1  block_type=mux  block_config=sysgen:Mux_config
  Out1 : Outport
  wires:
  In1/1 -> Mult/1
  AddSub/1 -> Mux/3, AddSub/2
  In2/1 -> Mult/2
  Mult/1 -> AddSub/1
  In3/1 -> Mux/1
  Mux/1 -> Out1/1
